simulink model "A2b"  (R2024a)
settings: Solver=ode113  StartTime=0.0  StopTime=100  RelTol=1e-3
settings Model: Creator=Flipper  LastModifiedBy=Flipper

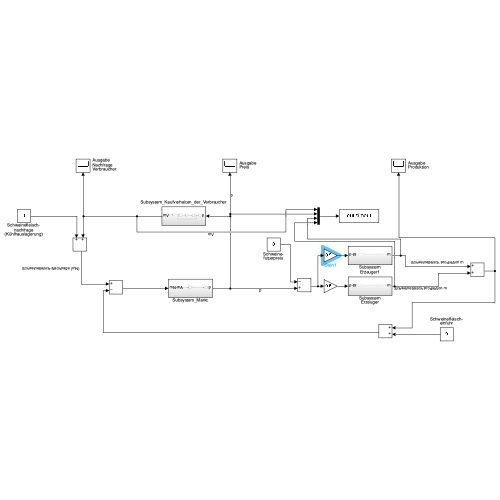
[thumbnail: Simulink's stored preview of the top-level diagram]
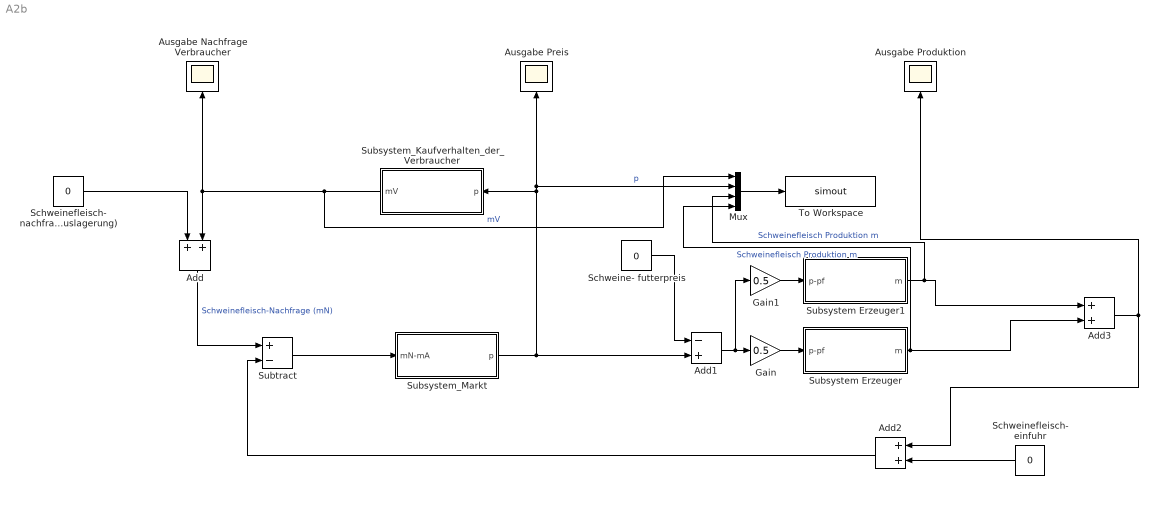
== system A2b ==
  Add : Sum
  Add1 : Sum  Inputs=-+
  Add2 : Sum
  Add3 : Sum
  Ausgabe Nachfrage Verbraucher : Scope
  Ausgabe Preis : Scope
  Ausgabe Produktion : Scope
  Gain : Gain  Gain=0.5
  Gain1 : Gain  Gain=0.5
  Mux : Mux
  Schweine- futterpreis : Constant  Value=0
  Schweinefleisch- einfuhr : Constant  Value=0
  Schweinefleisch- nachfrage (Kühlhauslagerung) : Constant  Value=0
  Subsystem Erzeuger : Subsystem
  Subsystem Erzeuger1 : Subsystem
  Subsystem_Kaufverhalten_der_Verbraucher : Subsystem
  Subsystem_Markt : Subsystem
  Subtract : Sum  Inputs=+-
  To Workspace : ToWorkspace  VariableName=simout  SaveFormat=Timeseries  SampleTime=-1
  wires:
  Subtract/1 -> Subsystem_Markt/1(mN-mA)
  Schweinefleisch- nachfrage (Kühlhauslagerung)/1 -> Add/1
  Schweinefleisch- einfuhr/1 -> Add2/2
  Schweine- futterpreis/1 -> Add1/1
  Add2/1 -> Subtract/2
  Subsystem_Kaufverhalten_der_Verbraucher/1(mV) -> Mux/1, Ausgabe Nachfrage Verbraucher/1, Add/2  "mV"
  Add/1 -> Subtract/1  "Schweinefleisch-Nachfrage (mN)"
  Subsystem_Markt/1(p) -> Ausgabe Preis/1, Mux/2, Subsystem_Kaufverhalten_der_Verbraucher/1(p), Add1/2  "p"
  Mux/1 -> To Workspace/1
  Gain/1 -> Subsystem Erzeuger/1(p-pf)
  Gain1/1 -> Subsystem Erzeuger1/1(p-pf)
  Add1/1 -> Gain1/1, Gain/1
  Subsystem Erzeuger1/1(m) -> Mux/3, Add3/1  "Schweinefleisch Produktion m"
  Subsystem Erzeuger/1(m) -> Mux/4, Add3/2  "Schweinefleisch Produktion m"
  Add3/1 -> Add2/1, Ausgabe Produktion/1

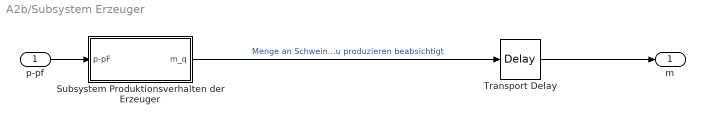
== system A2b/Subsystem Erzeuger ==
  p-pf : Inport
  Subsystem Produktionsverhalten der Erzeuger : Subsystem
  Transport Delay : TransportDelay  DelayTime=10
  m : Outport
  wires:
  p-pf/1 -> Subsystem Produktionsverhalten der Erzeuger/1(p-pF)
  Subsystem Produktionsverhalten der Erzeuger/1(m_q) -> Transport Delay/1  "Menge an Schweinefleisch, die der Erzeuger zu produzieren beabsichtigt"
  Transport Delay/1 -> m/1

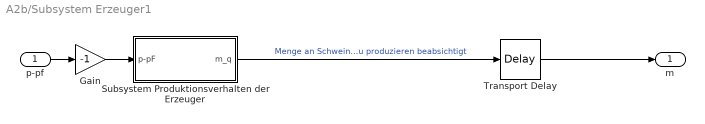
== system A2b/Subsystem Erzeuger1 ==
  p-pf : Inport
  Gain : Gain  Gain=-1
  Subsystem Produktionsverhalten der Erzeuger : Subsystem
  Transport Delay : TransportDelay  DelayTime=10
  m : Outport
  wires:
  p-pf/1 -> Gain/1
  Subsystem Produktionsverhalten der Erzeuger/1(m_q) -> Transport Delay/1  "Menge an Schweinefleisch, die der Erzeuger zu produzieren beabsichtigt"
  Transport Delay/1 -> m/1
  Gain/1 -> Subsystem Produktionsverhalten der Erzeuger/1(p-pF)

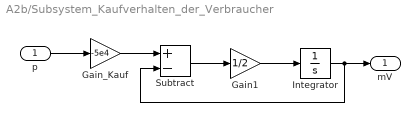
== system A2b/Subsystem_Kaufverhalten_der_Verbraucher ==
  p : Inport
  Gain1 : Gain  Gain=1/2
  Gain_Kauf : Gain  Gain=-5e4
  Integrator : Integrator  InitialCondition=-5e4
  Subtract : Sum  Inputs=+-
  mV : Outport
  wires:
  p/1 -> Gain_Kauf/1
  Gain_Kauf/1 -> Subtract/1
  Subtract/1 -> Gain1/1
  Gain1/1 -> Integrator/1
  Integrator/1 -> Subtract/2, mV/1

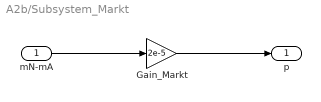
== system A2b/Subsystem_Markt ==
  mN-mA : Inport
  Gain_Markt : Gain  Gain=2e-5
  p : Outport
  wires:
  mN-mA/1 -> Gain_Markt/1
  Gain_Markt/1 -> p/1

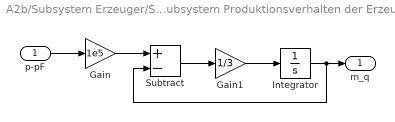
== system A2b/Subsystem Erzeuger/Subsystem Produktionsverhalten der Erzeuger ==
  p-pF : Inport
  Gain : Gain  Gain=1e5
  Gain1 : Gain  Gain=1/3
  Integrator : Integrator
  Subtract : Sum  Inputs=+-
  m_q : Outport
  wires:
  p-pF/1 -> Gain/1
  Gain/1 -> Subtract/1
  Subtract/1 -> Gain1/1
  Integrator/1 -> Subtract/2, m_q/1
  Gain1/1 -> Integrator/1

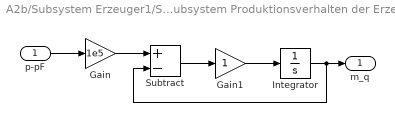
== system A2b/Subsystem Erzeuger1/Subsystem Produktionsverhalten der Erzeuger ==
  p-pF : Inport
  Gain : Gain  Gain=1e5
  Gain1 : Gain
  Integrator : Integrator
  Subtract : Sum  Inputs=+-
  m_q : Outport
  wires:
  p-pF/1 -> Gain/1
  Gain/1 -> Subtract/1
  Subtract/1 -> Gain1/1
  Integrator/1 -> Subtract/2, m_q/1
  Gain1/1 -> Integrator/1
